simulink model "flux_obs"  (R2025b)
settings: Solver=ode1  StartTime=0.0  StopTime=22  FixedStep=tc  MaxStep=tc  RelTol=1e-3
undefined symbols (not defined in the file): alpha_norm, beta_norm, gamma_norm, Lm_norm, Omega_s_bez, sigma_norm, ts_inv
settings Model: SimulationMode=accelerator  Creator=dbagn  LastModifiedBy=dbagn

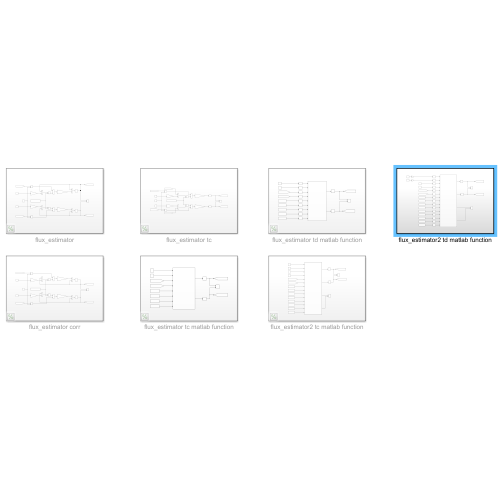
[thumbnail: Simulink's stored preview of the top-level diagram]
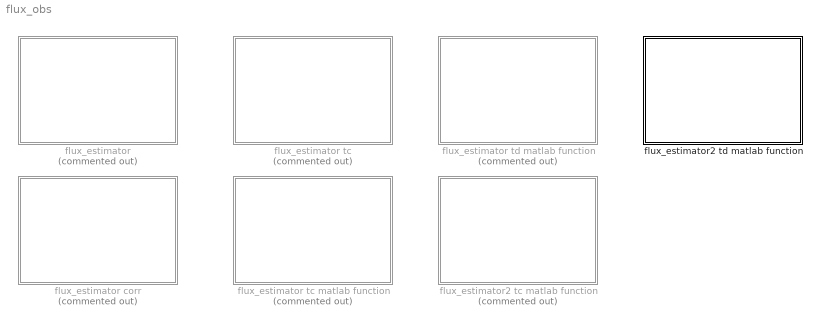
== system flux_obs ==
  flux_estimator : Subsystem  Commented=on
  flux_estimator corr : Subsystem  Commented=on
  flux_estimator tc : Subsystem  Commented=on
  flux_estimator tc matlab function : Subsystem  Commented=on
  flux_estimator td matlab function : Subsystem  Commented=on
  flux_estimator2 tc matlab function : Subsystem  Commented=on
  flux_estimator2 td matlab function : Subsystem

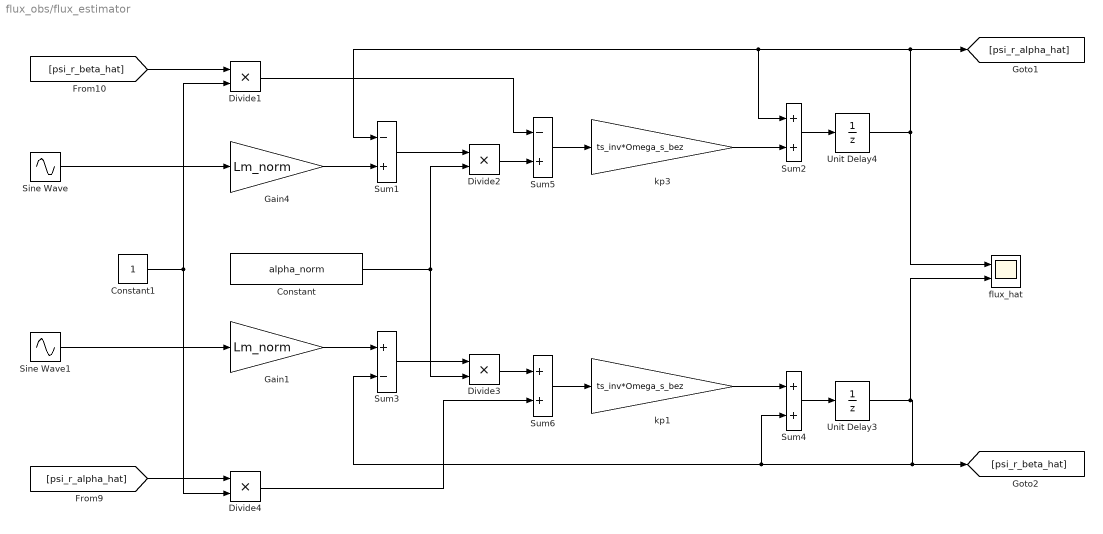
== system flux_obs/flux_estimator ==
  Constant : Constant  Value=alpha_norm
  Constant1 : Constant
  Divide{1..4} (4 alike) : Product
  Gain1 : Gain  Gain=Lm_norm
  Gain4 : Gain  Gain=Lm_norm
  Sine Wave : Sin  Amplitude=1/Lm_norm  Frequency=Omega_s_bez  Phase=pi/2  SampleTime=0
  Sine Wave1 : Sin  Amplitude=1/Lm_norm  Frequency=Omega_s_bez  SampleTime=0
  Sum1 : Sum  Inputs=-+  SaturateOnIntegerOverflow=on
  Sum2 : Sum  SaturateOnIntegerOverflow=on
  Sum3 : Sum  Inputs=+-  SaturateOnIntegerOverflow=on
  Sum4 : Sum  SaturateOnIntegerOverflow=on
  Sum5 : Sum  Inputs=-+  SaturateOnIntegerOverflow=on
  Sum6 : Sum  SaturateOnIntegerOverflow=on
  Unit Delay3 : UnitDelay  SampleTime=ts_inv  HasFrameUpgradeWarning=on
  Unit Delay4 : UnitDelay  SampleTime=ts_inv  HasFrameUpgradeWarning=on
  flux_hat : Scope  NumInputPorts=2
      settings: SampleTime=ts_inv  ActiveDisplayYMinimum=-5.4636482360346064E+16  ActiveDisplayYMaximum=5.3513191452893184E+16
  kp1 : Gain  Gain=ts_inv*Omega_s_bez  SaturateOnIntegerOverflow=on  OutDataTypeStr=Inherit: Same as input  ParamDataTypeStr=Inherit: Same as input
  kp3 : Gain  Gain=ts_inv*Omega_s_bez  SaturateOnIntegerOverflow=on  OutDataTypeStr=Inherit: Same as input  ParamDataTypeStr=Inherit: Same as input
  wires:
  Sum1/1 -> Divide2/1
  Sum3/1 -> Divide3/1
  Constant/1 -> Divide3/2, Divide2/2
  kp3/1 -> Sum2/2
  kp1/1 -> Sum4/1
  Sum2/1 -> Unit Delay4/1
  Sum4/1 -> Unit Delay3/1
  [psi_r_alpha_hat] -> Divide4/1
  [psi_r_beta_hat] -> Divide1/1
  Gain4/1 -> Sum1/2
  Divide2/1 -> Sum5/2
  Sum5/1 -> kp3/1
  Divide3/1 -> Sum6/1
  Sum6/1 -> kp1/1
  Divide4/1 -> Sum6/2
  Divide1/1 -> Sum5/1
  Unit Delay4/1 -> [psi_r_alpha_hat], Sum2/1, Sum1/1, flux_hat/1
  Unit Delay3/1 -> flux_hat/2, [psi_r_beta_hat], Sum3/2, Sum4/2
  Constant1/1 -> Divide4/2, Divide1/2
  Sine Wave/1 -> Gain4/1
  Sine Wave1/1 -> Gain1/1
  Gain1/1 -> Sum3/1

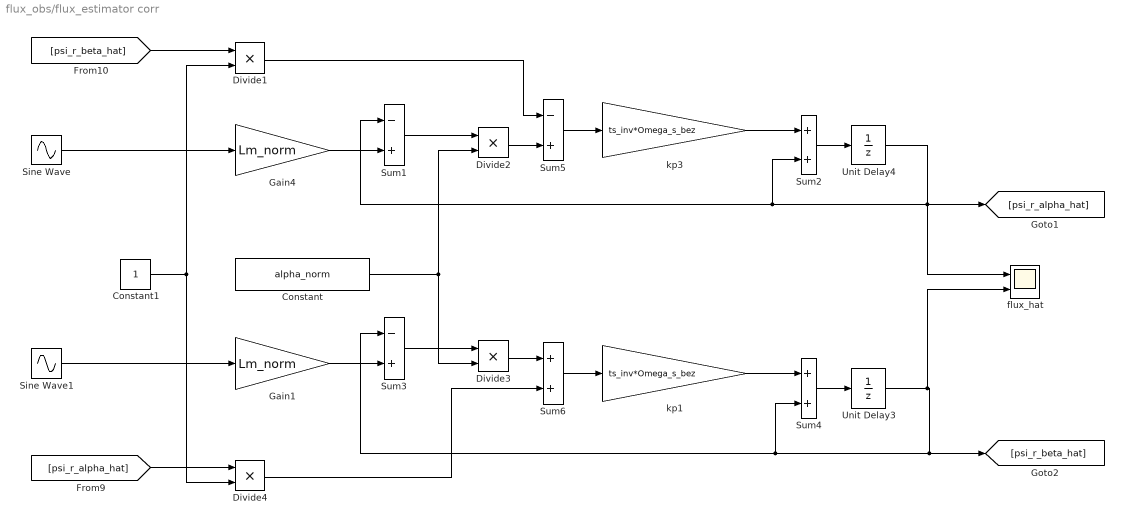
== system flux_obs/flux_estimator corr ==
  Constant : Constant  Value=alpha_norm
  Constant1 : Constant
  Divide{1..4} (4 alike) : Product
  Gain1 : Gain  Gain=Lm_norm
  Gain4 : Gain  Gain=Lm_norm
  Sine Wave : Sin  Frequency=2*pi*50  SampleTime=0
  Sine Wave1 : Sin  Frequency=2*pi*50  Phase=pi/2  SampleTime=0
  Sum1 : Sum  Inputs=-+  SaturateOnIntegerOverflow=on
  Sum2 : Sum  SaturateOnIntegerOverflow=on
  Sum3 : Sum  Inputs=-+  SaturateOnIntegerOverflow=on
  Sum4 : Sum  SaturateOnIntegerOverflow=on
  Sum5 : Sum  Inputs=-+  SaturateOnIntegerOverflow=on
  Sum6 : Sum  SaturateOnIntegerOverflow=on
  Unit Delay3 : UnitDelay  SampleTime=ts_inv  HasFrameUpgradeWarning=on
  Unit Delay4 : UnitDelay  InitialCondition=1  SampleTime=ts_inv  HasFrameUpgradeWarning=on
  flux_hat : Scope  NumInputPorts=2
      settings: SampleTime=ts_inv/100  ActiveDisplayYMinimum=-1.2378480386690085  ActiveDisplayYMaximum=1.2499397313298413
  kp1 : Gain  Gain=ts_inv*Omega_s_bez  SaturateOnIntegerOverflow=on  OutDataTypeStr=Inherit: Same as input  ParamDataTypeStr=Inherit: Same as input
  kp3 : Gain  Gain=ts_inv*Omega_s_bez  SaturateOnIntegerOverflow=on  OutDataTypeStr=Inherit: Same as input  ParamDataTypeStr=Inherit: Same as input
  wires:
  Sine Wave1/1 -> Gain1/1
  Sine Wave/1 -> Gain4/1
  Constant1/1 -> Divide4/2, Divide1/2
  Unit Delay3/1 -> Sum3/1, Sum4/2, [psi_r_beta_hat], flux_hat/2
  Unit Delay4/1 -> Sum1/1, Sum2/2, [psi_r_alpha_hat], flux_hat/1
  Divide1/1 -> Sum5/1
  Divide4/1 -> Sum6/2
  Sum6/1 -> kp1/1
  Divide3/1 -> Sum6/1
  Sum5/1 -> kp3/1
  Divide2/1 -> Sum5/2
  Gain1/1 -> Sum3/2
  Gain4/1 -> Sum1/2
  [psi_r_beta_hat] -> Divide1/1
  [psi_r_alpha_hat] -> Divide4/1
  Sum4/1 -> Unit Delay3/1
  Sum2/1 -> Unit Delay4/1
  kp1/1 -> Sum4/1
  kp3/1 -> Sum2/1
  Constant/1 -> Divide3/2, Divide2/2
  Sum3/1 -> Divide3/1
  Sum1/1 -> Divide2/1

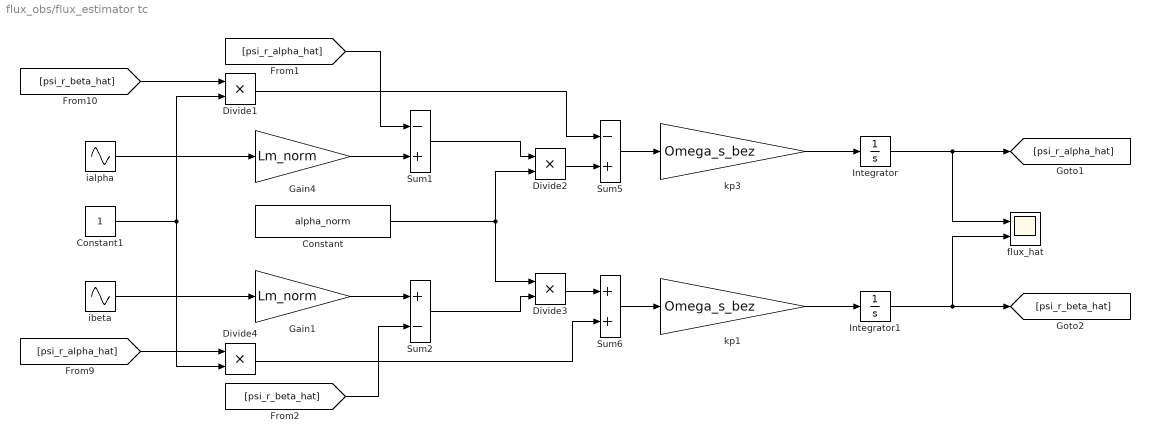
== system flux_obs/flux_estimator tc ==
  Constant : Constant  Value=alpha_norm
  Constant1 : Constant
  Divide{1..4} (4 alike) : Product
  Gain1 : Gain  Gain=Lm_norm
  Gain4 : Gain  Gain=Lm_norm
  Integrator : Integrator
  Integrator1 : Integrator
  Sum1 : Sum  Inputs=-+  SaturateOnIntegerOverflow=on
  Sum2 : Sum  Inputs=+-  SaturateOnIntegerOverflow=on
  Sum5 : Sum  Inputs=-+  SaturateOnIntegerOverflow=on
  Sum6 : Sum  SaturateOnIntegerOverflow=on
  flux_hat : Scope  NumInputPorts=2
      settings: SampleTime=ts_inv  ActiveDisplayYMinimum=-1.2499997972695536  ActiveDisplayYMaximum=1.2499997953368243
  ialpha : Sin  Amplitude=1/Lm_norm  Frequency=Omega_s_bez  Phase=pi/2  SampleTime=0
  ibeta : Sin  Amplitude=1/Lm_norm  Frequency=Omega_s_bez  SampleTime=0
  kp1 : Gain  Gain=Omega_s_bez  SaturateOnIntegerOverflow=on  OutDataTypeStr=Inherit: Same as input  ParamDataTypeStr=Inherit: Same as input
  kp3 : Gain  Gain=Omega_s_bez  SaturateOnIntegerOverflow=on  OutDataTypeStr=Inherit: Same as input  ParamDataTypeStr=Inherit: Same as input
  wires:
  ibeta/1 -> Gain1/1
  ialpha/1 -> Gain4/1
  Constant1/1 -> Divide4/2, Divide1/2
  Divide1/1 -> Sum5/1
  Divide4/1 -> Sum6/2
  Sum6/1 -> kp1/1
  Divide3/1 -> Sum6/1
  Sum5/1 -> kp3/1
  Divide2/1 -> Sum5/2
  [psi_r_beta_hat] -> Divide1/1
  [psi_r_alpha_hat] -> Divide4/1
  kp1/1 -> Integrator1/1
  kp3/1 -> Integrator/1
  Constant/1 -> Divide3/1, Divide2/2
  Gain4/1 -> Sum1/2
  Sum1/1 -> Divide2/1
  Gain1/1 -> Sum2/1
  Sum2/1 -> Divide3/2
  [psi_r_alpha_hat] -> Sum1/1
  [psi_r_beta_hat] -> Sum2/2
  Integrator/1 -> flux_hat/1, [psi_r_alpha_hat]
  Integrator1/1 -> [psi_r_beta_hat], flux_hat/2

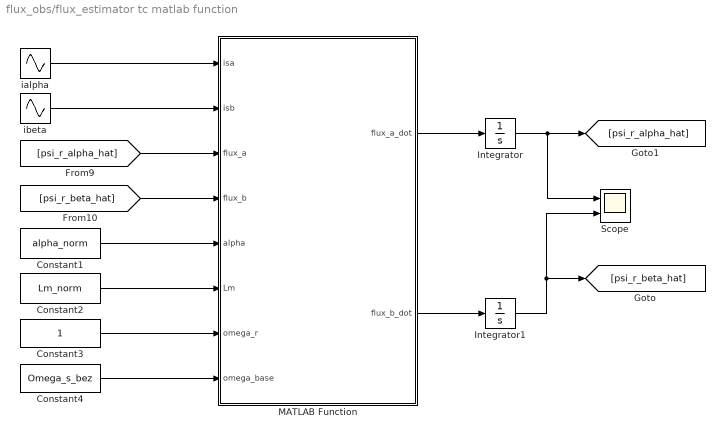
== system flux_obs/flux_estimator tc matlab function ==
  Constant1 : Constant  Value=alpha_norm
  Constant2 : Constant  Value=Lm_norm
  Constant3 : Constant
  Constant4 : Constant  Value=Omega_s_bez
  Integrator : Integrator
  Integrator1 : Integrator
  MATLAB Function : MATLAB Function  TreatAsAtomicUnit=on
  Scope : Scope  NumInputPorts=2
      settings: SampleTime=tc  ActiveDisplayYMinimum=-1.0806468952029975  ActiveDisplayYMaximum=1.0795597144902858
  ialpha : Sin  Amplitude=1/Lm_norm  Frequency=Omega_s_bez  Phase=pi/2  SampleTime=0
  ibeta : Sin  Amplitude=1/Lm_norm  Frequency=Omega_s_bez  SampleTime=0
  wires:
  MATLAB Function/1(flux_a_dot) -> Integrator/1
  MATLAB Function/2(flux_b_dot) -> Integrator1/1
  Integrator1/1 -> Scope/2, [psi_r_beta_hat]
  Integrator/1 -> [psi_r_alpha_hat], Scope/1
  [psi_r_beta_hat] -> MATLAB Function/4(flux_b)
  [psi_r_alpha_hat] -> MATLAB Function/3(flux_a)
  ialpha/1 -> MATLAB Function/1(isa)
  ibeta/1 -> MATLAB Function/2(isb)
  Constant1/1 -> MATLAB Function/5(alpha)
  Constant2/1 -> MATLAB Function/6(Lm)
  Constant3/1 -> MATLAB Function/7(omega_r)
  Constant4/1 -> MATLAB Function/8(omega_base)

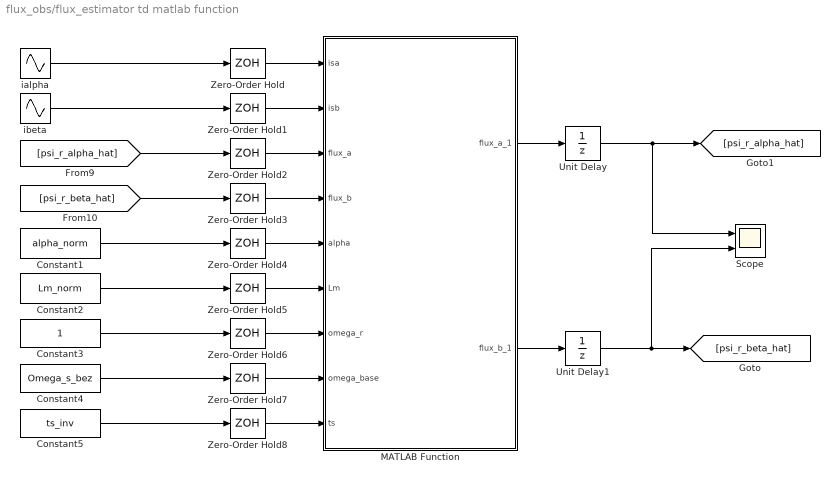
== system flux_obs/flux_estimator td matlab function ==
  Constant1 : Constant  Value=alpha_norm
  Constant2 : Constant  Value=Lm_norm
  Constant3 : Constant
  Constant4 : Constant  Value=Omega_s_bez
  Constant5 : Constant  Value=ts_inv
  MATLAB Function : MATLAB Function  TreatAsAtomicUnit=on  SystemSampleTime=ts_inv
  Scope : Scope  NumInputPorts=2
      settings: SampleTime=tc  ActiveDisplayYMinimum=-5.9658567331502432E-5  ActiveDisplayYMaximum=5.9848044555494216E-5
  Unit Delay : UnitDelay  SampleTime=ts_inv  HasFrameUpgradeWarning=on
  Unit Delay1 : UnitDelay  SampleTime=ts_inv  HasFrameUpgradeWarning=on
  Zero-Order Hold{,1..8} (9 alike) : ZeroOrderHold  SampleTime=ts_inv
  ialpha : Sin  Amplitude=1/Lm_norm  Frequency=Omega_s_bez  Phase=pi/2  SampleTime=0
  ibeta : Sin  Amplitude=1/Lm_norm  Frequency=Omega_s_bez  SampleTime=0
  wires:
  Constant4/1 -> Zero-Order Hold7/1
  Constant2/1 -> Zero-Order Hold5/1
  Constant1/1 -> Zero-Order Hold4/1
  ibeta/1 -> Zero-Order Hold1/1
  ialpha/1 -> Zero-Order Hold/1
  [psi_r_alpha_hat] -> Zero-Order Hold2/1
  [psi_r_beta_hat] -> Zero-Order Hold3/1
  Unit Delay/1 -> [psi_r_alpha_hat], Scope/1
  MATLAB Function/2(flux_b_1) -> Unit Delay1/1
  MATLAB Function/1(flux_a_1) -> Unit Delay/1
  Unit Delay1/1 -> Scope/2, [psi_r_beta_hat]
  Constant5/1 -> Zero-Order Hold8/1
  Zero-Order Hold/1 -> MATLAB Function/1(isa)
  Zero-Order Hold1/1 -> MATLAB Function/2(isb)
  Zero-Order Hold2/1 -> MATLAB Function/3(flux_a)
  Zero-Order Hold3/1 -> MATLAB Function/4(flux_b)
  Zero-Order Hold4/1 -> MATLAB Function/5(alpha)
  Zero-Order Hold5/1 -> MATLAB Function/6(Lm)
  Zero-Order Hold6/1 -> MATLAB Function/7(omega_r)
  Zero-Order Hold7/1 -> MATLAB Function/8(omega_base)
  Zero-Order Hold8/1 -> MATLAB Function/9(ts)
  Constant3/1 -> Zero-Order Hold6/1

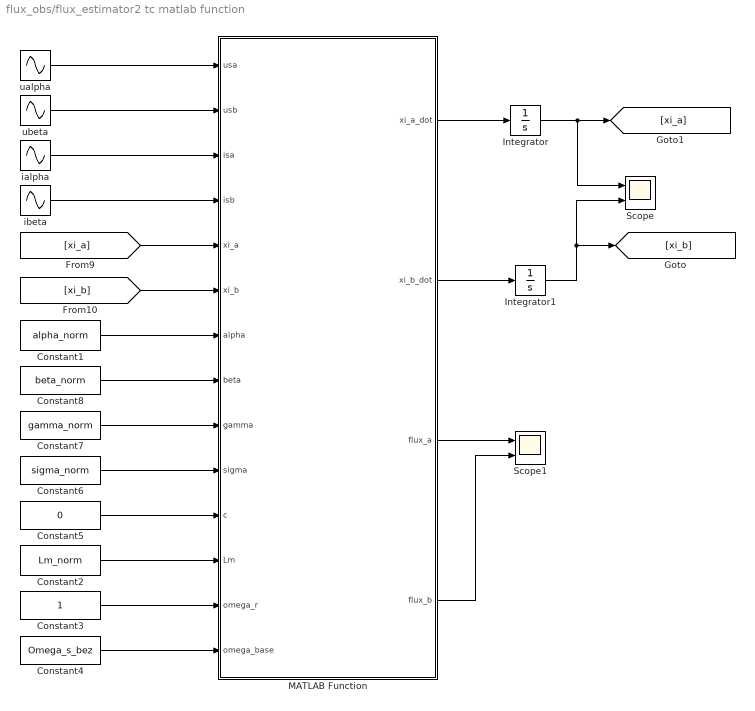
== system flux_obs/flux_estimator2 tc matlab function ==
  Constant1 : Constant  Value=alpha_norm
  Constant2 : Constant  Value=Lm_norm
  Constant3 : Constant
  Constant4 : Constant  Value=Omega_s_bez
  Constant5 : Constant  Value=0
  Constant6 : Constant  Value=sigma_norm
  Constant7 : Constant  Value=gamma_norm
  Constant8 : Constant  Value=beta_norm
  Integrator : Integrator
  Integrator1 : Integrator
  MATLAB Function : MATLAB Function  TreatAsAtomicUnit=on
  Scope : Scope  NumInputPorts=2
      settings: ActiveDisplayYMinimum=-1.2499999933469741  ActiveDisplayYMaximum=1.2499999933528545
  Scope1 : Scope  NumInputPorts=2
      settings: ActiveDisplayYMinimum=-1.2499999933469741  ActiveDisplayYMaximum=1.2499999933528545  DataLoggingVariableName=ScopeData2
  ialpha : Sin  Amplitude=1/Lm_norm  Frequency=Omega_s_bez  Phase=pi/2  SampleTime=0
  ibeta : Sin  Amplitude=1/Lm_norm  Frequency=Omega_s_bez  SampleTime=0
  ualpha : Sin  Amplitude=1/Lm_norm  Frequency=Omega_s_bez  Phase=pi/2  SampleTime=0
  ubeta : Sin  Amplitude=1/Lm_norm  Frequency=Omega_s_bez  SampleTime=0
  wires:
  Constant4/1 -> MATLAB Function/14(omega_base)
  Constant3/1 -> MATLAB Function/13(omega_r)
  Constant2/1 -> MATLAB Function/12(Lm)
  Constant1/1 -> MATLAB Function/7(alpha)
  ibeta/1 -> MATLAB Function/4(isb)
  ialpha/1 -> MATLAB Function/3(isa)
  [xi_a] -> MATLAB Function/5(xi_a)
  [xi_b] -> MATLAB Function/6(xi_b)
  Integrator/1 -> Scope/1, [xi_a]
  Integrator1/1 -> [xi_b], Scope/2
  MATLAB Function/2(xi_b_dot) -> Integrator1/1
  MATLAB Function/1(xi_a_dot) -> Integrator/1
  MATLAB Function/3(flux_a) -> Scope1/1
  MATLAB Function/4(flux_b) -> Scope1/2
  Constant5/1 -> MATLAB Function/11(c)
  Constant6/1 -> MATLAB Function/10(sigma)
  Constant7/1 -> MATLAB Function/9(gamma)
  Constant8/1 -> MATLAB Function/8(beta)
  ubeta/1 -> MATLAB Function/2(usb)
  ualpha/1 -> MATLAB Function/1(usa)

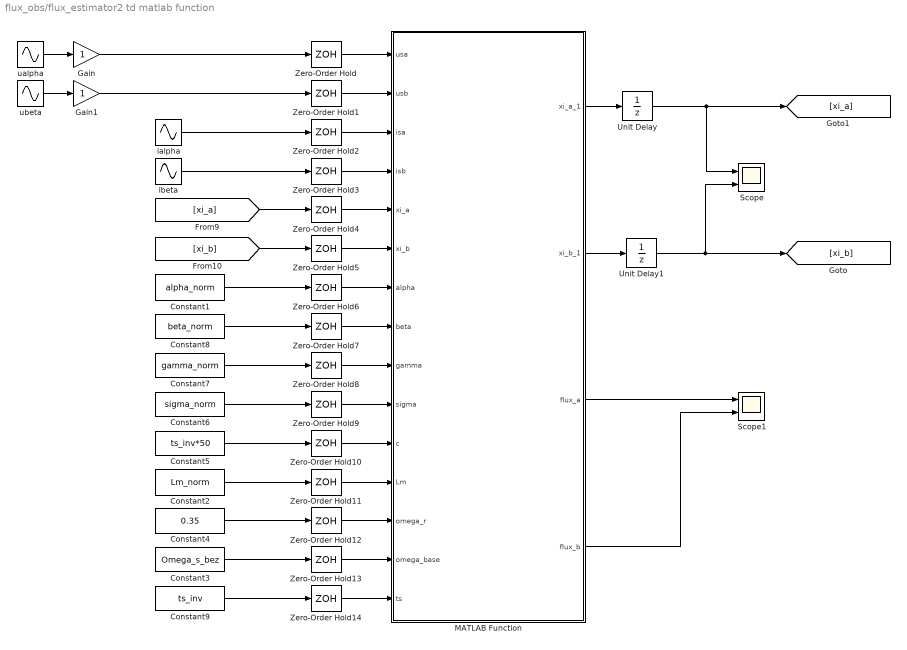
== system flux_obs/flux_estimator2 td matlab function ==
  Constant1 : Constant  Value=alpha_norm
  Constant2 : Constant  Value=Lm_norm
  Constant3 : Constant  Value=Omega_s_bez
  Constant4 : Constant  Value=0.35
  Constant5 : Constant  Value=ts_inv*50
  Constant6 : Constant  Value=sigma_norm
  Constant7 : Constant  Value=gamma_norm
  Constant8 : Constant  Value=beta_norm
  Constant9 : Constant  Value=ts_inv
  Gain : Gain
  Gain1 : Gain
  MATLAB Function : MATLAB Function  TreatAsAtomicUnit=on  SystemSampleTime=ts_inv
  Scope : Scope  NumInputPorts=2
      settings: ActiveDisplayYMinimum=-2.7591129741175164  ActiveDisplayYMaximum=2.8548618898890794
  Scope1 : Scope  NumInputPorts=2
      settings: ActiveDisplayYMinimum=-2.76666447365536  ActiveDisplayYMaximum=2.8272437388021476  DataLoggingVariableName=ScopeData2
  Unit Delay : UnitDelay  SampleTime=ts_inv  HasFrameUpgradeWarning=on
  Unit Delay1 : UnitDelay  SampleTime=ts_inv  HasFrameUpgradeWarning=on
  Zero-Order Hold{,1..14} (15 alike) : ZeroOrderHold  SampleTime=ts_inv
  ialpha : Sin  Amplitude=1/Lm_norm  Frequency=Omega_s_bez*0.35  Phase=pi/2  SampleTime=0
  ibeta : Sin  Amplitude=1/Lm_norm  Frequency=Omega_s_bez*0.35  SampleTime=0
  ualpha : Sin  Amplitude=1/Lm_norm  Frequency=Omega_s_bez*0.35  Phase=pi/2  SampleTime=0
  ubeta : Sin  Amplitude=1/Lm_norm  Frequency=Omega_s_bez*0.35  SampleTime=0
  wires:
  ualpha/1 -> Gain/1
  Constant8/1 -> Zero-Order Hold7/1
  Constant7/1 -> Zero-Order Hold8/1
  Constant6/1 -> Zero-Order Hold9/1
  Constant5/1 -> Zero-Order Hold10/1
  MATLAB Function/4(flux_b) -> Scope1/2
  MATLAB Function/3(flux_a) -> Scope1/1
  [xi_b] -> Zero-Order Hold5/1
  [xi_a] -> Zero-Order Hold4/1
  ialpha/1 -> Zero-Order Hold2/1
  ibeta/1 -> Zero-Order Hold3/1
  Constant1/1 -> Zero-Order Hold6/1
  Constant2/1 -> Zero-Order Hold11/1
  Constant9/1 -> Zero-Order Hold14/1
  Zero-Order Hold/1 -> MATLAB Function/1(usa)
  Zero-Order Hold1/1 -> MATLAB Function/2(usb)
  Zero-Order Hold2/1 -> MATLAB Function/3(isa)
  Zero-Order Hold3/1 -> MATLAB Function/4(isb)
  Zero-Order Hold4/1 -> MATLAB Function/5(xi_a)
  Zero-Order Hold5/1 -> MATLAB Function/6(xi_b)
  Zero-Order Hold6/1 -> MATLAB Function/7(alpha)
  Zero-Order Hold7/1 -> MATLAB Function/8(beta)
  Zero-Order Hold8/1 -> MATLAB Function/9(gamma)
  Zero-Order Hold9/1 -> MATLAB Function/10(sigma)
  Zero-Order Hold10/1 -> MATLAB Function/11(c)
  Zero-Order Hold11/1 -> MATLAB Function/12(Lm)
  Zero-Order Hold12/1 -> MATLAB Function/13(omega_r)
  Zero-Order Hold13/1 -> MATLAB Function/14(omega_base)
  Zero-Order Hold14/1 -> MATLAB Function/15(ts)
  Constant3/1 -> Zero-Order Hold13/1
  Constant4/1 -> Zero-Order Hold12/1
  Unit Delay/1 -> [xi_a], Scope/1
  Unit Delay1/1 -> Scope/2, [xi_b]
  MATLAB Function/1(xi_a_1) -> Unit Delay/1
  MATLAB Function/2(xi_b_1) -> Unit Delay1/1
  Gain/1 -> Zero-Order Hold/1
  ubeta/1 -> Gain1/1
  Gain1/1 -> Zero-Order Hold1/1

== matlab function flux_obs/flux_estimator td matlab function/MATLAB Function ==
  data: isa input; flux_a_1 output; isb input; flux_a input; flux_b input; alpha input; Lm input; omega_r input; flux_b_1 output; omega_base input; ts input
function [flux_a_1, flux_b_1] = flux_obs(isa, isb, flux_a, flux_b, ...
    alpha, Lm, omega_r, omega_base,  ts)

    flux_a_1 = flux_a + ts*omega_base*(-alpha*flux_a - omega_r*flux_b + alpha*Lm*isa);
    flux_b_1 = flux_b + ts*omega_base*(-alpha*flux_b + omega_r*flux_a + alpha*Lm*isb);

== matlab function flux_obs/flux_estimator tc matlab function/MATLAB Function ==
  data: isa input; flux_a_dot output; isb input; flux_a input; flux_b input; alpha input; Lm input; omega_r input; flux_b_dot output; omega_base input
function [flux_a_dot, flux_b_dot] = flux_obs(isa, isb, flux_a, flux_b, ...
    alpha, Lm, omega_r, omega_base)

    flux_a_dot = omega_base*(-alpha*flux_a - omega_r*flux_b + alpha*Lm*isa);
    flux_b_dot = omega_base*(-alpha*flux_b + omega_r*flux_a + alpha*Lm*isb);

== matlab function flux_obs/flux_estimator2 tc matlab function/MATLAB Function ==
  data: usa input; usb input; isa input; xi_a_dot output; isb input; xi_a input; xi_b input; alpha input; beta input; gamma input; sigma input; c input; Lm input; omega_r input; xi_b_dot output; omega_base input; flux_a output; flux_b output
function [xi_a_dot, xi_b_dot, flux_a, flux_b] = flux_obs(usa, usb, isa, isb, xi_a, xi_b, ...
    alpha, beta, gamma, sigma, c, Lm, omega_r, omega_base)

    
    xi_a_dot = omega_base*(-alpha*(1+c*beta)*xi_a - omega_r*(1+c*beta)*xi_b + ...
        ((alpha*Lm + c*gamma) - alpha*c*(1 + c*beta))*isa - omega_r*c*(1 + c*beta)*isb - ...
        c/sigma*usa);

    xi_b_dot = omega_base*(-alpha*(1+c*beta)*xi_b + omega_r*(1+c*beta)*xi_a + ...
        ((alpha*Lm + c*gamma) - alpha*c*(1 + c*beta))*isb + omega_r*c*(1 + c*beta)*isa - ...
        c/sigma*usb);

    flux_a = c*isa+xi_a;
    flux_b = c*isb+xi_b;

== matlab function flux_obs/flux_estimator2 td matlab function/MATLAB Function ==
  data: usa input; usb input; isa input; xi_a_1 output; isb input; xi_a input; xi_b input; alpha input; beta input; gamma input; sigma input; c input; Lm input; omega_r input; xi_b_1 output; omega_base input; flux_a output; flux_b output; ts input
function [xi_a_1, xi_b_1, flux_a, flux_b] = flux_obs(usa, usb, isa, isb, xi_a, xi_b, ...
    alpha, beta, gamma, sigma, c, Lm, omega_r, omega_base, ts)
 
    xi_a_1 = xi_a + ts*omega_base*(-alpha*(1+c*beta)*xi_a - omega_r*(1+c*beta)*xi_b + ...
        ((alpha*Lm + c*gamma) - alpha*c*(1 + c*beta))*isa - omega_r*c*(1 + c*beta)*isb - ...
        c/sigma*usa);

    xi_b_1 = xi_b + ts*omega_base*(-alpha*(1+c*beta)*xi_b + omega_r*(1+c*beta)*xi_a + ...
        ((alpha*Lm + c*gamma) - alpha*c*(1 + c*beta))*isb + omega_r*c*(1 + c*beta)*isa - ...
        c/sigma*usb);

    flux_a = c*isa + xi_a;
    flux_b = c*isb + xi_b;
